simulink model "A1Q4"  (R2021b)
settings: Solver=VariableStepAuto  StartTime=0.0  StopTime=10.0  RelTol=1e-3
libraries: fl_lib x14, nesl_utility x11, ee_lib x2, spspowerguiLib x1
settings Model: Creator=hansr  LastModifiedBy=hansr

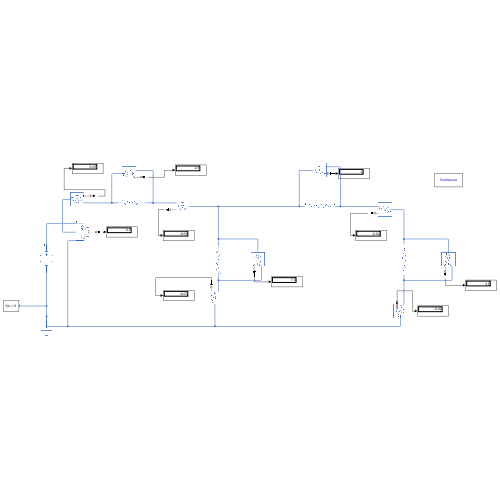
[thumbnail: Simulink's stored preview of the top-level diagram]
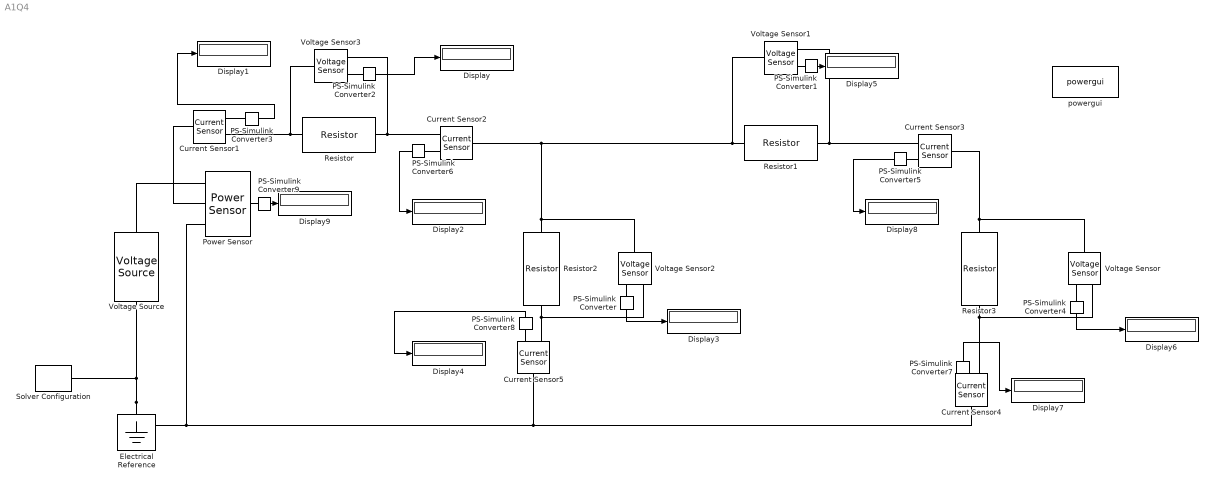
== system A1Q4 ==
  Current Sensor{1..5} (5 alike) : fl_lib/Electrical/Electrical Sensors/Current Sensor
  Display{,1..9} (10 alike) : Display
  Electrical Reference : fl_lib/Electrical/Electrical Elements/Electrical Reference
  PS-Simulink Converter{,1..9} (10 alike) : nesl_utility/PS-Simulink Converter  PhysicalDomain=network_engine_domain  SubClassName=ps_output  LeftPortType=input  RightPortType=output  PseudoPeriodic=off  Frequencies=[]  Unit=inherit  AffineConversion=off
      settings: SourceProductBaseCode=PW,SS
  Power Sensor : ee_lib/Sensors & Transducers/Power Sensor  measurement_type=1  averaging_period=1e-4 s
      settings: SourceProductBaseCode=PS
  Resistor : fl_lib/Electrical/Electrical Elements/Resistor  R=50 Ohm  i_specify=off  i_priority=None  i=0 A  i_nominal_specify=off  i_nominal_unit=A  i_nominal_value=1  v_specify=off  v_priority=None  v=0 V  v_nominal_specify=off  v_nominal_unit=V  v_nominal_value=1
  Resistor1 : fl_lib/Electrical/Electrical Elements/Resistor  R=200 Ohm  i_specify=off  i_priority=None  i=0 A  i_nominal_specify=off  i_nominal_unit=A  i_nominal_value=1  v_specify=off  v_priority=None  v=0 V  v_nominal_specify=off  v_nominal_unit=V  v_nominal_value=1
  Resistor2 : fl_lib/Electrical/Electrical Elements/Resistor  R=250 Ohm  i_specify=off  i_priority=None  i=0 A  i_nominal_specify=off  i_nominal_unit=A  i_nominal_value=1  v_specify=off  v_priority=None  v=0 V  v_nominal_specify=off  v_nominal_unit=V  v_nominal_value=1
  Resistor3 : fl_lib/Electrical/Electrical Elements/Resistor  R=175 Ohm  i_specify=off  i_priority=None  i=0 A  i_nominal_specify=off  i_nominal_unit=A  i_nominal_value=1  v_specify=off  v_priority=None  v=0 V  v_nominal_specify=off  v_nominal_unit=V  v_nominal_value=1
  Solver Configuration : nesl_utility/Solver Configuration  PhysicalDomain=network_engine_domain  SubClassName=solver  LeftPortType=input  RightPortType=generic  Tones=[]  Harmonics=[]  SimulateNoise=off  Profile=off  UseLocalSampling=off  EnableSwitchedLinearOptims=on  FrequencyDomain=off  UseCCode=off  RelTol=0.001  AbsTol=1e-06  MinStep=1e-09  ToWorkspace=off  RevertToSquareIcSolve=off  NumHomotopyIterations=100  PhasorMode=off  PhasorModeNumHarmonics=1  DoDC=off  ResidualTolerance=1e-09  UseLocalSolver=off  LocalSolverChoice=NE_BACKWARD_EULER_ADVANCER  LocalSolverSampleTime=0.001  DoFixedCost=off  MaxNonlinIter=3  MaxModeIter=2  ComputeImpulses=off  ImpulseIterations=2  LinearAlgebra=auto  EquationFormulation=NE_TIME_EF  DelaysMemoryBudget=1024  AutomaticFiltering=on  FilteringTimeConstant=0.001  PartitionStorageMethod=AS_NEEDED  PartitionMemoryBudget=1024  PartitionMethod=ROBUST
      settings: SourceProductBaseCode=PW,SS
  Voltage Sensor{,1..3} (4 alike) : fl_lib/Electrical/Electrical Sensors/Voltage Sensor
  Voltage Source : ee_lib/Sources/Voltage Source  dc_voltage=10 V  ac_voltage=0 V  ac_shift=0 rad  ac_frequency=60 Hz  noise_mode=0  PSD=0 V^2/Hz  repeatability=1  auto_seed=711455876  user_seed=0  sample_time=1e-3 s  i_specify=off  i_priority=None  i=0 A  i_nominal_specify=off  i_nominal_unit=A  i_nominal_value=1  v_specify=off  v_priority=None  v=0 V  v_nominal_specify=off  v_nominal_unit=V  v_nominal_value=1
  powergui : spspowerguiLib/powergui  Priority=1  SimulationMode=Continuous  SampleTime=50e-6  frequency=60  Iterations=50  frequencyindice=60  Pbase=100e6  ErrMax=1e-4  UnitsV=kV  UnitsW=MW  buscounter=0  FunctionMessages=off  echomessages=off  EnableUseOfTLC=off  CurrentSourceSwitches=off  DisableSnubberDevices=off  DisableRonSwitches=off  DisableVfSwitches=off  DisplayEquations=off  AutomaticDiscreteSolvers=off  SolverType=Tustin/Backward Euler (TBE)  Interpol=off  ExternalGateDelay=off  methode=off  Ts=100  x0status=blocks  SPID=on  SwTol=0  HookPort=off  NonlinearTolerance=1e-4  nMaxIteration=100  ContinueOnMaxIteration=off  RestoreLinks=warning  ResistiveCurrentMeasurement=off  Frange=[0:2:500]  Ylog=off  Xlog=on  ShowGrid=off  save=off  variable=ZData  structure=0  ZoomFFT=off  StartTime=0.0  cycles=1  DisplayStyle=1  fundamental=60  FreqAxis=off  MaxFrequency=1000  frequencyindicesteady=1  RmsSteady=1  display=off
  wires:
  PS-Simulink Converter2/1 -> Display/1
  PS-Simulink Converter3/1 -> Display1/1
  PS-Simulink Converter6/1 -> Display2/1
  PS-Simulink Converter/1 -> Display3/1
  PS-Simulink Converter8/1 -> Display4/1
  PS-Simulink Converter1/1 -> Display5/1
  PS-Simulink Converter4/1 -> Display6/1
  PS-Simulink Converter7/1 -> Display7/1
  PS-Simulink Converter5/1 -> Display8/1
  PS-Simulink Converter9/1 -> Display9/1
  connections:
  Voltage Sensor/LConn1 -- Current Sensor3/LConn1 -- Resistor3/LConn1
  Voltage Sensor/RConn2 -- Current Sensor4/RConn2 -- Resistor3/RConn1
  Voltage Sensor1/LConn1 -- Voltage Sensor2/LConn1 -- Resistor2/LConn1 -- Current Sensor2/LConn1 -- Resistor1/LConn1
  Voltage Sensor1/RConn2 -- Current Sensor3/RConn2 -- Resistor1/RConn1
  Voltage Sensor2/RConn2 -- Current Sensor5/RConn2 -- Resistor2/RConn1
  Voltage Sensor3/LConn1 -- Current Sensor1/RConn2 -- Resistor/LConn1
  Voltage Sensor3/RConn2 -- Current Sensor2/RConn2 -- Resistor/RConn1
  Voltage Source/RConn1 -- Solver Configuration/RConn1 -- Power Sensor/LConn3 -- Current Sensor5/LConn1 -- Current Sensor4/LConn1 -- Electrical Reference/LConn1
  PS-Simulink Converter1/LConn1 -- Voltage Sensor1/RConn1
  PS-Simulink Converter2/LConn1 -- Voltage Sensor3/RConn1
  PS-Simulink Converter3/LConn1 -- Current Sensor1/RConn1
  PS-Simulink Converter/LConn1 -- Voltage Sensor2/RConn1
  PS-Simulink Converter4/LConn1 -- Voltage Sensor/RConn1
  PS-Simulink Converter5/LConn1 -- Current Sensor3/RConn1
  PS-Simulink Converter6/LConn1 -- Current Sensor2/RConn1
  PS-Simulink Converter7/LConn1 -- Current Sensor4/RConn1
  PS-Simulink Converter8/LConn1 -- Current Sensor5/RConn1
  Voltage Source/LConn1 -- Power Sensor/LConn1
  Power Sensor/LConn2 -- Current Sensor1/LConn1
  PS-Simulink Converter9/LConn1 -- Power Sensor/RConn1
